simulink model "tno_cpi"  (R2025b)
settings: Solver=VariableStepAuto  StartTime=0.0  StopTime=10.0  RelTol=1e-3
libraries: Delft_Tyre_dtlib x1, Delft_Tyre_sm1glib x1
settings Model: Creator=niekv  LastModifiedBy=niekv

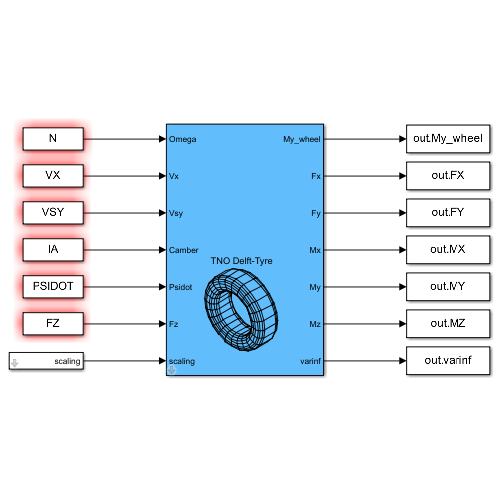
[thumbnail: Simulink's stored preview of the top-level diagram]
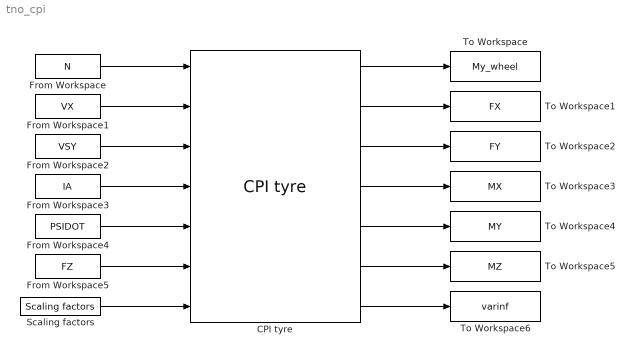
== system tno_cpi ==
  CPI tyre : Delft_Tyre_dtlib/Simulink/CPI tyre  Tag=CPI tyre  idtyre=1  tpfname=[]  side_mode=(1xxx) left  dyn_mode=(xx0x) steady-state  mf_mode=(xxx0) none  use_mode=1e8  disp_debug=off
  From Workspace : FromWorkspace  VariableName=N
  From Workspace1 : FromWorkspace  VariableName=VX
  From Workspace2 : FromWorkspace  VariableName=VSY
  From Workspace3 : FromWorkspace  VariableName=IA
  From Workspace4 : FromWorkspace  VariableName=PSIDOT
  From Workspace5 : FromWorkspace  VariableName=FZ
  Scaling factors : Delft_Tyre_sm1glib/SimMechanics 1G/Scaling factors  Tag=Scaling factors  LMUX=1  LKX=1  LMUY=1  LKY=1  LKYC=1  LTR=1  LKZC=1
  To Workspace : ToWorkspace  VariableName=My_wheel  SaveFormat=Timeseries  SampleTime=-1
  To Workspace1 : ToWorkspace  VariableName=FX  SaveFormat=Timeseries  SampleTime=-1
  To Workspace2 : ToWorkspace  VariableName=FY  SaveFormat=Timeseries  SampleTime=-1
  To Workspace3 : ToWorkspace  VariableName=MX  SaveFormat=Timeseries  SampleTime=-1
  To Workspace4 : ToWorkspace  VariableName=MY  SaveFormat=Timeseries  SampleTime=-1
  To Workspace5 : ToWorkspace  VariableName=MZ  SaveFormat=Timeseries  SampleTime=-1
  To Workspace6 : ToWorkspace  VariableName=varinf  SaveFormat=Timeseries  SampleTime=-1
  wires:
  From Workspace/1 -> CPI tyre/1
  From Workspace1/1 -> CPI tyre/2
  From Workspace2/1 -> CPI tyre/3
  From Workspace3/1 -> CPI tyre/4
  From Workspace4/1 -> CPI tyre/5
  From Workspace5/1 -> CPI tyre/6
  Scaling factors/1 -> CPI tyre/7
  CPI tyre/7 -> To Workspace6/1
  CPI tyre/6 -> To Workspace5/1
  CPI tyre/5 -> To Workspace4/1
  CPI tyre/4 -> To Workspace3/1
  CPI tyre/3 -> To Workspace2/1
  CPI tyre/2 -> To Workspace1/1
  CPI tyre/1 -> To Workspace/1
